simulink model "ModelBlocks"  (R2023a)
settings: Solver=ode45  StartTime=0.0  StopTime=10000  RelTol=1e-30
model workspace (MAT data in the model file):
  N_p0 = 5
  N_v0 = 0
  N_w0 = 0
  t_ion = 0
  t_p = 12
  t_pump = 32
  t_release = 5
  t_retention = 2
libraries: simulink x1
settings Model: ParameterArgumentNames=N_p0,N_v0,N_w0,t_ion,t_p,t_pump,t_release,t_retention  Creator=levsi  LastModifiedBy=levsi
settings DataIOCC: ReturnWorkspaceOutputs=off

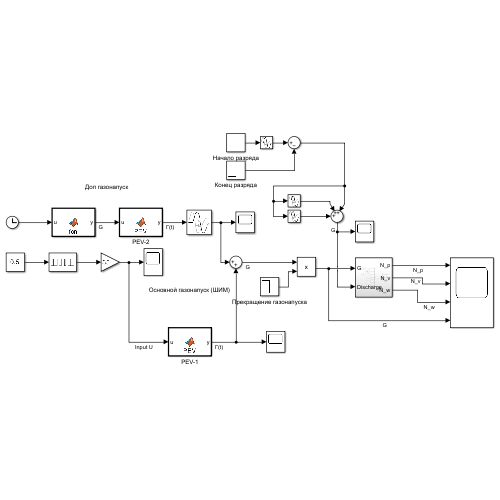
[thumbnail: Simulink's stored preview of the top-level diagram]
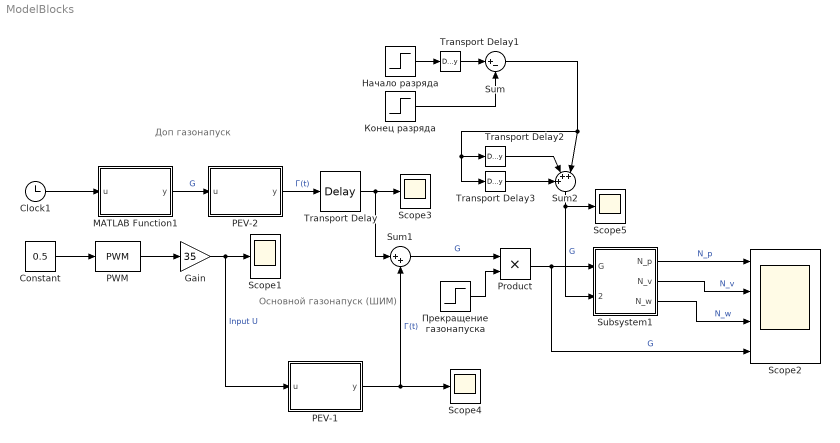
== system ModelBlocks ==
  note: Доп газонапуск
  note: Основной газонапуск (ШИМ)
  Clock1 : Clock
  Constant : Constant  Value=0.5
  Gain : Gain  Gain=35
  MATLAB Function1 : MATLAB Function  TreatAsAtomicUnit=on
  PEV-1 : MATLAB Function  TreatAsAtomicUnit=on
  PEV-2 : MATLAB Function  TreatAsAtomicUnit=on
  PWM : simulink/Discontinuities/PWM  DisableCoverage=on  Period=0.5  InitialDelay=0  DisallowZeroDutyCycle=off  RunAtFixedTimeIntervals=off  SampleTime=0.1
  Product : Product
  Scope{1,3..5} (4 alike) : Scope
  Scope2 : Scope  NumInputPorts=4
  Subsystem1 : Subsystem
  Sum : Sum  Inputs=|+-
  Sum1 : Sum  Inputs=|++
  Sum2 : Sum  Inputs=+++|
  Transport Delay : TransportDelay  DelayTime=25
  Transport Delay1 : TransportDelay  DelayTime=0.12
  Transport Delay2 : TransportDelay  DelayTime=1000
  Transport Delay3 : TransportDelay  DelayTime=5000
  Конец разряда : Step  Time=428  SampleTime=0
  Начало разряда : Step  Time=427.1  SampleTime=0
  Прекращение газонапуска : Step  Time=500  Before=1  After=0  SampleTime=0
  wires:
  Subsystem1/3(N_w) -> Scope2/3  "N_w"
  Subsystem1/2(N_v) -> Scope2/2  "N_v"
  Subsystem1/1(N_p) -> Scope2/1  "N_p"
  Clock1/1 -> MATLAB Function1/1(u)
  Constant/1 -> PWM/1
  Gain/1 -> PEV-1/1(u), Scope1/1  "Input U"
  PEV-1/1(y) -> Scope4/1, Sum1/2  "Г(t)"
  PWM/1 -> Gain/1
  PEV-2/1(y) -> Transport Delay/1  "Г(t)"
  MATLAB Function1/1(y) -> PEV-2/1(u)  "G"
  Конец разряда/1 -> Sum/2
  Sum/1 -> Sum2/3, Transport Delay3/1, Transport Delay2/1
  Transport Delay/1 -> Sum1/1, Scope3/1
  Sum1/1 -> Product/1  "G"
  Прекращение газонапуска/1 -> Product/2
  Product/1 -> Scope2/4, Subsystem1/1(G)  "G"
  Transport Delay1/1 -> Sum/1
  Начало разряда/1 -> Transport Delay1/1
  Sum2/1 -> Subsystem1/2(Discharge), Scope5/1  "G"
  Transport Delay2/1 -> Sum2/2
  Transport Delay3/1 -> Sum2/1

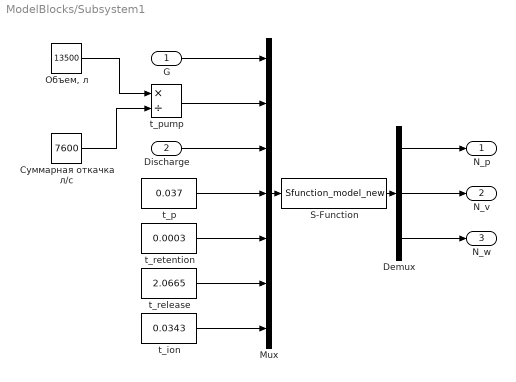
== system ModelBlocks/Subsystem1 ==
  G : Inport
  Discharge : Inport  Port=2
  Demux : Demux  Outputs=3
  Mux : Mux  Inputs=7
  S-Function : S-Function  FunctionName=Sfunction_model_new  Parameters=0, 5.7e18, 1.9460e22  SFunctionDeploymentMode=off  EnableBusSupport=off
  t_ion : Constant  Value=0.0343
  t_p : Constant  Value=0.037
  t_pump : Product  Inputs=*/
  t_release : Constant  Value=2.0665
  t_retention : Constant  Value=0.0003
  "Объем, л" : Constant  Value=13500
  Суммарная откачка л/с : Constant  Value=7600
  N_p : Outport
  N_v : Outport  Port=2
  N_w : Outport  Port=3
  wires:
  Demux/1 -> N_p/1
  S-Function/1 -> Demux/1
  Demux/2 -> N_v/1
  Demux/3 -> N_w/1
  G/1 -> Mux/1
  Mux/1 -> S-Function/1
  "Объем, л"/1 -> t_pump/1
  t_pump/1 -> Mux/2
  Суммарная откачка л/с/1 -> t_pump/2
  Discharge/1 -> Mux/3
  t_p/1 -> Mux/4
  t_retention/1 -> Mux/5
  t_release/1 -> Mux/6
  t_ion/1 -> Mux/7

== matlab function ModelBlocks/PEV-1 ==
  data: u input; y output
function y = PEV(u)
    y_vals = [0, 18, 28, 42, 62, 80, 100, 123, 154, 180, 200, 232, 259, 280, 300, 323, 346, 360, 400, 433, 450, 478, 500, 538, 552, 580, 600, 635, 668, 700, 729, 750, 770, 800, 839, 870, 900, 930, 958, 988, 1000, 1050, 1100];
    x_vals = [20, 32, 35, 40, 44.8, 48.2, 50, 52.2, 54.8, 56.5, 57.5, 60, 61.7, 62.8, 63.9, 65, 66.1, 67.5, 70, 71, 72, 74, 75, 76.5, 78, 80, 82, 83, 85, 87, 88, 90, 90.8, 91.8, 93, 94.5, 96.2, 97.2, 98, 98.2, 98.5, 98.8, 99];
    if (u >= x_vals(1))
        Gase = interp1(x_vals, y_vals, u);
    else
        Gase = 0;
    end
    y = Gase * 0.0980665*6.02e23/(60*8.31*300);
end

== matlab function ModelBlocks/PEV-2 ==
  data: u input; y output
function y = PEV(u)
    y_vals = [0, 18, 28, 42, 62, 80, 100, 123, 154, 180, 200, 232, 259, 280, 300, 323, 346, 360, 400, 433, 450, 478, 500, 538, 552, 580, 600, 635, 668, 700, 729, 750, 770, 800, 839, 870, 900, 930, 958, 988, 1000, 1050, 1100];
    x_vals = [20, 32, 35, 40, 44.8, 48.2, 50, 52.2, 54.8, 56.5, 57.5, 60, 61.7, 62.8, 63.9, 65, 66.1, 67.5, 70, 71, 72, 74, 75, 76.5, 78, 80, 82, 83, 85, 87, 88, 90, 90.8, 91.8, 93, 94.5, 96.2, 97.2, 98, 98.2, 98.5, 98.8, 99];
    if (u >= x_vals(1))
        Gase = interp1(x_vals, y_vals, u);
    else
        Gase = 0;
    end
    y = Gase * 0.0980665*6.02e23/(60*8.31*300);
end

== matlab function ModelBlocks/MATLAB Function1 ==
  data: u input; y output
function y = fcn(u)

if (u>=2.1) && (u<2.5)
    y = 60;
elseif (u>=2.5) && (u<3)
    y = 55;
else
    y = 0;
end

end
